simulink model "dspafxf_win32"  (Simulink 5.0)
settings: Solver=FixedStepDiscrete  StartTime=0.0  StopTime=3.928  RelTol=1e-3
PreLoadFcn:
  | load dspafxf;
undefined symbols (not defined in the file or in its folder): fs_afxf
libraries: dspwin32 x2, dspsrcs4 x2, dspmtrx3 x1, dspsigops x1
settings Model: CovMetricSettings=d  Creator=don  LastModifiedBy=mristivo  ExtModeTrigMode=oneshot  ExtModeArmWhenConnect=off  SaveTime=off  SaveOutput=off  LimitDataPoints=off  SingleTaskRateTransMsg=error  IntegerOverflowMsg=none  BlockReductionOpt=off  BooleanDataType=off  ZeroCross=off  RTWOptions=-aRollThreshold=2

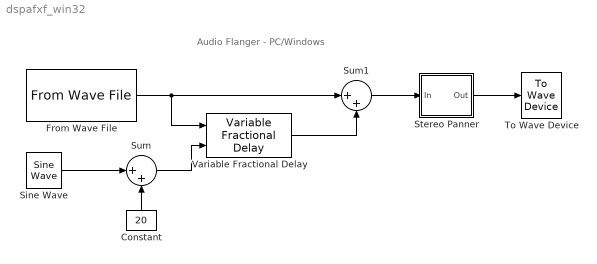
== system dspafxf_win32 ==
  note: Audio Flanger - PC/Windows
  Constant : Constant  Orientation=up  Value=20
  From Wave File : dspwin32/From Wave File  FileName=dspafxf.wav  SamplesPerFrame=128  MinBufSize=512  dType=Double
  Sine Wave : dspsrcs4/Sine Wave  Amplitude=15  Frequency=1/3.394  Phase=pi/4  SampleMode=Discrete  OutComplex=Real  CompMethod=Trigonometric fcn  TableSize=Speed  SampleTime=1/fs_afxf  SamplesPerFrame=128  dataType=double  wordLen=16  udDataType=sfix(16)  fracBitsMode=Best precision  numFracBits=14  ResetState=Restart at time zero
  Stereo Panner : Subsystem
  Sum : Sum  Inputs=|++  SaturateOnIntegerOverflow=on  InputSameDT=on
  Sum1 : Sum  Inputs=|++  SaturateOnIntegerOverflow=on  InputSameDT=on
  To Wave Device : dspwin32/To Wave Device  bufDuration=3  initDelay=0.1  useDefaultDevice=on  enable24Bit=off
  Variable Fractional Delay : dspsigops/Variable Fractional Delay  mode=FIR Interpolation  dmax=100  L=8  R=10  alpha=0.5  ic=0
  wires:
  Constant/1 -> Sum/2
  Sine Wave/1 -> Sum/1
  From Wave File/1 -> Variable Fractional Delay/1, Sum1/1
  Sum/1 -> Variable Fractional Delay/2
  Variable Fractional Delay/1 -> Sum1/2
  Sum1/1 -> Stereo Panner/1(In)
  Stereo Panner/1(Out) -> To Wave Device/1

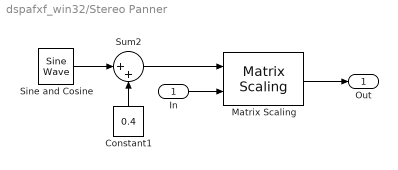
== system dspafxf_win32/Stereo Panner ==
  In : Inport
  Constant1 : Constant  Orientation=up  Value=0.4
  Matrix Scaling : dspmtrx3/Matrix Scaling  mode=Scale Rows (D*A)
  Sine and Cosine : dspsrcs4/Sine Wave  Amplitude=0.4  Frequency=1/3.934 * 1.5  Phase=[-pi/2 pi/2]  SampleMode=Discrete  OutComplex=Real  CompMethod=Trigonometric fcn  TableSize=Speed  SampleTime=1/fs_afxf  SamplesPerFrame=128  dataType=double  wordLen=16  udDataType=sfix(16)  fracBitsMode=Best precision  numFracBits=14  ResetState=Restart at time zero
  Sum2 : Sum  Inputs=|++  SaturateOnIntegerOverflow=on  InputSameDT=on
  Out : Outport
  wires:
  Matrix Scaling/1 -> Out/1
  Constant1/1 -> Sum2/2
  Sine and Cosine/1 -> Sum2/1
  Sum2/1 -> Matrix Scaling/1
  In/1 -> Matrix Scaling/2
